simulink model "discrete_control_with_noise"  (Simulink 7.4)
settings: Solver=ode45  StartTime=0.0  StopTime=30.0  RelTol=1e-3
values from neighbouring files (symbols this model uses):
  f1 = (I_y-I_z)/I_x    [quadrocopter_param.m]
  f2 = rot.J_z/I_x    [quadrocopter_param.m]
  f3 = (I_z-I_x)/I_y    [quadrocopter_param.m]
  f4 = rot.J_z/I_y    [quadrocopter_param.m]
  f5 = (I_x-I_y)/I_z    [quadrocopter_param.m]
  g = 9.81    [quadrocopter_param.m]
  I_x = elec.I_x+bat.I_x+2*boom.I_1x+2*boom.I_1y+2*mot.I_1x+2*mot.I_1y+                             2*rot.I_1x+2*rot.I_1y    [quadrocopter_param.m]
  I_y = elec.I_y+bat.I_y+2*boom.I_1x+2*boom.I_1y+2*mot.I_1x+2*mot.I_1y+                             2*rot.I_1x+2*rot.I_1y    [quadrocopter_param.m]
  I_z = elec.I_z+bat.I_z+4*boom.I_1z+4*mot.I_1z+4*rot.I_1z    [quadrocopter_param.m]
  phi0 = 0.15    [Quadrocopter_control_Driver.m]    (also in calc_stability.m = 0; control_two_angles_Driver.m; control_two_angles_and_yawrate_Driver.m; discrete_control_phi_theta_rpsi_Driver.m)
  r_psi0 = 0    [Quadrocopter_control_Driver.m]    (also in calc_stability.m; control_two_angles_Driver.m = 0.01; control_two_angles_and_yawrate_Driver.m = 0.01; discrete_control_phi_theta_rpsi_Driver.m = 0.01)
  theta0 = 0.15    [Quadrocopter_control_Driver.m]    (also in calc_stability.m = 0; control_two_angles_Driver.m; control_two_angles_and_yawrate_Driver.m; discrete_control_phi_theta_rpsi_Driver.m)
  Ts = 0.005    [quadrocopter_param.m]
undefined symbols (not defined in the file or in its folder): boom
libraries: Copter_Library x5
settings Model: Creator=Robert  LastModifiedBy=roczit00

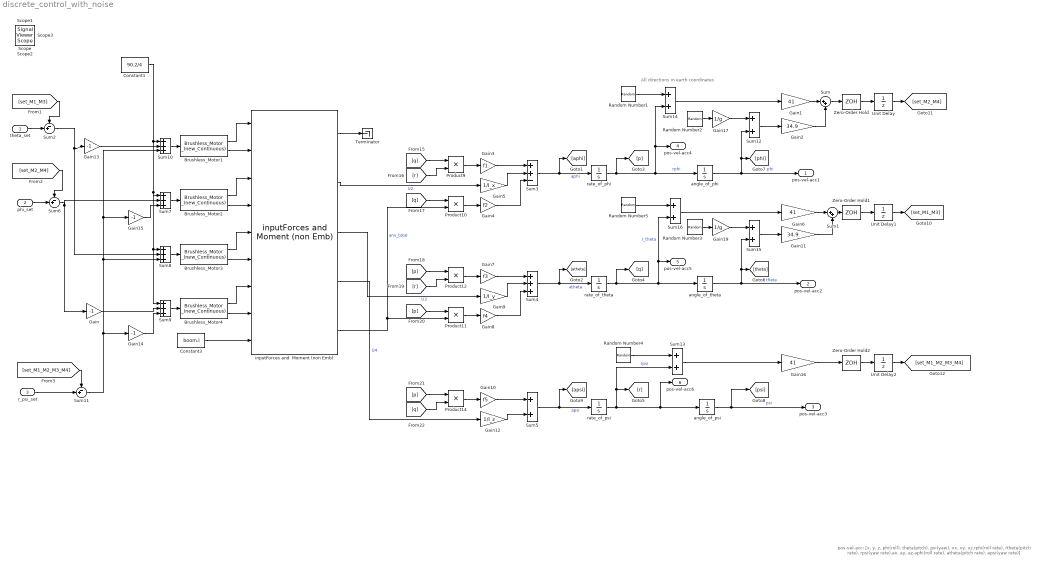
== system discrete_control_with_noise ==
  note: pos-vel-acc: [x, y, z, phi(roll), theta(pitch), psi(yaw), vx, vy, vz,rphi(roll rate), rtheta(pitch rate), rpsi(yaw rate),ax, ay, az,aphi(roll rate), atheta(pitch rate), apsi(yaw rate)]
  note: All directions in earth coordinates
  theta_set : Inport  OutDataType=fixdt(1, 16)  OutScaling=2^0
  phi_set : Inport  Port=2  OutDataType=fixdt(1, 16)  OutScaling=2^0
  r_psi_set : Inport  Port=3  OutDataType=fixdt(1, 16)  OutScaling=2^0
  Brushless_Motor{1..4} (4 alike) : Copter_Library/Brushless_Motor _(new_Continuous)  SystemSampleTime=-1  M_error=1
  Constant1 : Constant  Value=90.2/4  OutDataType=fixdt(1, 16)  OutScaling=2^0
  Constant3 : Constant  Value=boom.l  OutDataType=fixdt(1, 16)  OutScaling=2^0
  Gain{,13..15} (4 alike) : Gain  Gain=-1  ParameterDataType=fixdt(1, 16)  ParameterScaling=2^0  OutDataType=fixdt(1, 16)  OutScaling=2^0
  Gain1 : Gain  Gain=41  ParameterDataType=fixdt(1, 16)  ParameterScaling=2^0  OutDataType=fixdt(1, 16)  OutScaling=2^0
  Gain10 : Gain  Gain=f5  ParameterDataType=fixdt(1, 16)  ParameterScaling=2^0  OutDataType=fixdt(1, 16)  OutScaling=2^0
  Gain11 : Gain  Gain=34.9  ParameterDataType=fixdt(1, 16)  ParameterScaling=2^0  OutDataType=fixdt(1, 16)  OutScaling=2^0
  Gain12 : Gain  Gain=1/I_z  ParameterDataType=fixdt(1, 16)  ParameterScaling=2^0  OutDataType=fixdt(1, 16)  OutScaling=2^0
  Gain16 : Gain  Gain=41  ParameterDataType=fixdt(1, 16)  ParameterScaling=2^0  OutDataType=fixdt(1, 16)  OutScaling=2^0
  Gain17 : Gain  Gain=1/g  ParameterDataType=fixdt(1, 16)  ParameterScaling=2^0  OutDataType=fixdt(1, 16)  OutScaling=2^0
  Gain19 : Gain  Gain=1/g  ParameterDataType=fixdt(1, 16)  ParameterScaling=2^0  OutDataType=fixdt(1, 16)  OutScaling=2^0
  Gain2 : Gain  Gain=34.9  ParameterDataType=fixdt(1, 16)  ParameterScaling=2^0  OutDataType=fixdt(1, 16)  OutScaling=2^0
  Gain3 : Gain  Gain=f1  ParameterDataType=fixdt(1, 16)  ParameterScaling=2^0  OutDataType=fixdt(1, 16)  OutScaling=2^0
  Gain4 : Gain  Gain=f2  ParameterDataType=fixdt(1, 16)  ParameterScaling=2^0  OutDataType=fixdt(1, 16)  OutScaling=2^0
  Gain5 : Gain  Gain=1/I_x  ParameterDataType=fixdt(1, 16)  ParameterScaling=2^0  OutDataType=fixdt(1, 16)  OutScaling=2^0
  Gain6 : Gain  Gain=41  ParameterDataType=fixdt(1, 16)  ParameterScaling=2^0  OutDataType=fixdt(1, 16)  OutScaling=2^0
  Gain7 : Gain  Gain=f3  ParameterDataType=fixdt(1, 16)  ParameterScaling=2^0  OutDataType=fixdt(1, 16)  OutScaling=2^0
  Gain8 : Gain  Gain=f4  ParameterDataType=fixdt(1, 16)  ParameterScaling=2^0  OutDataType=fixdt(1, 16)  OutScaling=2^0
  Gain9 : Gain  Gain=1/I_y  ParameterDataType=fixdt(1, 16)  ParameterScaling=2^0  OutDataType=fixdt(1, 16)  OutScaling=2^0
  Product{9..12,14} (5 alike) : Product  OutDataType=fixdt(1, 16)  OutScaling=2^0  RndMeth=Zero
  Random Number1 : RandomNumber  Variance=3.0462e-8  Seed=45632  SampleTime=0.01
  Random Number2 : RandomNumber  Variance=0.0003  Seed=4564  SampleTime=0.01
  Random Number3 : RandomNumber  Variance=0.0003  Seed=676  SampleTime=Ts
  Random Number4 : RandomNumber  Variance=3.0462e-8  Seed=1634  SampleTime=0.01
  Random Number5 : RandomNumber  Variance=3.0462e-8  Seed=4731  SampleTime=0.01
  Sum : Sum  Inputs=|++  OutDataType=fixdt(1, 16)  OutScaling=2^0
  Sum1 : Sum  Inputs=|++  OutDataType=fixdt(1, 16)  OutScaling=2^0
  Sum{4,7..10} (5 alike) : Sum  Inputs=+++  OutDataType=fixdt(1, 16)  OutScaling=2^0
  Sum11 : Sum  Inputs=-+|  OutDataType=fixdt(1, 16)  OutScaling=2^0
  Sum{5,12..16} (6 alike) : Sum  OutDataType=fixdt(1, 16)  OutScaling=2^0
  Sum2 : Sum  Inputs=-+|  OutDataType=fixdt(1, 16)  OutScaling=2^0
  Sum3 : Sum  Inputs=++-  OutDataType=fixdt(1, 16)  OutScaling=2^0
  Sum6 : Sum  Inputs=-+|  OutDataType=fixdt(1, 16)  OutScaling=2^0
  Terminator : Terminator
  Unit Delay : UnitDelay  SampleTime=Ts
  Unit Delay1 : UnitDelay  SampleTime=Ts
  Unit Delay2 : UnitDelay  SampleTime=Ts
  Zero-Order Hold : ZeroOrderHold  SampleTime=Ts
  Zero-Order Hold1 : ZeroOrderHold  SampleTime=Ts
  Zero-Order Hold2 : ZeroOrderHold  SampleTime=Ts
  angle_of_phi : Integrator  InitialCondition=phi0
  angle_of_psi : Integrator
  angle_of_theta : Integrator  InitialCondition=theta0
  inputForces and  Moment (non Emb) : Copter_Library/inputForces and  Moment (non Emb)  SystemSampleTime=-1
  rate_of_phi : Integrator
  rate_of_psi : Integrator  InitialCondition=r_psi0
  rate_of_theta : Integrator
  pos-vel-acc1 : Outport  OutDataType=fixdt(1, 16)  OutScaling=2^0
  pos-vel-acc2 : Outport  Port=2  OutDataType=fixdt(1, 16)  OutScaling=2^0
  pos-vel-acc3 : Outport  Port=3  OutDataType=fixdt(1, 16)  OutScaling=2^0
  pos-vel-acc4 : Outport  Port=4  OutDataType=fixdt(1, 16)  OutScaling=2^0
  pos-vel-acc5 : Outport  Port=5  OutDataType=fixdt(1, 16)  OutScaling=2^0
  pos-vel-acc6 : Outport  Port=6  OutDataType=fixdt(1, 16)  OutScaling=2^0
  Scope : SignalViewerScope  IOType=viewer  ZoomMode=yonly  RefreshTime=0.035000
      settings: ShowLegends=on
  Scope1 : SignalViewerScope  IOType=viewer  ZoomMode=yonly  RefreshTime=0.035000
      settings: ShowLegends=on
  Scope2 : SignalViewerScope  IOType=viewer  ZoomMode=yonly  RefreshTime=0.035000
      settings: ShowLegends=on  SaveName=ScopeData2
  Scope3 : SignalViewerScope  IOType=viewer  ZoomMode=xonly  RefreshTime=0.035000
      settings: ShowLegends=on  SaveName=ScopeData3
  wires:
  Constant3/1 -> inputForces and  Moment (non Emb)/9
  Sum5/1 -> [apsi], rate_of_psi/1  "apsi"
  inputForces and  Moment (non Emb)/4 -> Gain12/1  "U4"
  Gain12/1 -> Sum5/2
  Gain10/1 -> Sum5/1
  Product14/1 -> Gain10/1
  [q] -> Product14/2
  [p] -> Product14/1
  Sum4/1 -> [atheta], rate_of_theta/1  "atheta"
  inputForces and  Moment (non Emb)/3 -> Gain9/1  "U3"
  Gain8/1 -> Sum4/3
  Gain9/1 -> Sum4/2
  Product11/1 -> Gain8/1
  [p] -> Product11/1
  Gain7/1 -> Sum4/1
  Product12/1 -> Gain7/1
  [r] -> Product12/2
  [p] -> Product12/1
  Sum3/1 -> [aphi], rate_of_phi/1  "aphi"
  Gain4/1 -> Sum3/3
  Gain5/1 -> Sum3/2
  inputForces and  Moment (non Emb)/2 -> Gain5/1  "U2"
  Product10/1 -> Gain4/1
  [q] -> Product10/1
  Gain3/1 -> Sum3/1
  Product9/1 -> Gain3/1
  [r] -> Product9/2
  [q] -> Product9/1
  inputForces and  Moment (non Emb)/5 -> Product11/2, Product10/2  "anv_total"
  angle_of_phi/1 -> pos-vel-acc1/1, [phi], Sum12/2  "phi"
  angle_of_theta/1 -> pos-vel-acc2/1, [theta], Sum15/2  "theta"
  angle_of_psi/1 -> [psi], pos-vel-acc3/1  "psi"
  rate_of_phi/1 -> [p], angle_of_phi/1, pos-vel-acc4/1, Sum14/2  "rphi"
  rate_of_theta/1 -> angle_of_theta/1, pos-vel-acc5/1, Sum16/2, [q]  "r_theta"
  rate_of_psi/1 -> angle_of_psi/1, pos-vel-acc6/1, [r], Sum13/2  "rpsi"
  Brushless_Motor1/1 -> inputForces and  Moment (non Emb)/1
  Brushless_Motor1/2 -> inputForces and  Moment (non Emb)/2
  Brushless_Motor2/1 -> inputForces and  Moment (non Emb)/3
  Brushless_Motor2/2 -> inputForces and  Moment (non Emb)/4
  Brushless_Motor3/1 -> inputForces and  Moment (non Emb)/5
  Brushless_Motor3/2 -> inputForces and  Moment (non Emb)/6
  Brushless_Motor4/1 -> inputForces and  Moment (non Emb)/7
  Brushless_Motor4/2 -> inputForces and  Moment (non Emb)/8
  Gain1/1 -> Sum/1
  Gain2/1 -> Sum/2
  Gain6/1 -> Sum1/1
  Gain11/1 -> Sum1/2
  [set_M1_M3] -> Sum2/1
  theta_set/1 -> Sum2/2
  Sum2/1 -> Gain13/1, Sum8/2
  phi_set/1 -> Sum6/2
  [set_M2_M4] -> Sum6/1
  Sum6/1 -> Gain/1, Sum7/2
  inputForces and  Moment (non Emb)/1 -> Terminator/1
  Sum9/1 -> Brushless_Motor4/1
  Sum8/1 -> Brushless_Motor3/1
  Sum7/1 -> Brushless_Motor2/1
  Sum10/1 -> Brushless_Motor1/1
  Constant1/1 -> Sum10/1, Sum7/1, Sum8/1, Sum9/1
  Gain13/1 -> Sum10/2
  Gain/1 -> Sum9/2
  r_psi_set/1 -> Sum11/2
  [set_M1_M2_M3_M4] -> Sum11/1
  Gain15/1 -> Sum7/3
  Sum11/1 -> Gain14/1, Sum8/3, Gain15/1, Sum10/3
  Gain14/1 -> Sum9/3
  Sum/1 -> Zero-Order Hold/1
  Sum1/1 -> Zero-Order Hold1/1
  Gain16/1 -> Zero-Order Hold2/1
  Zero-Order Hold2/1 -> Unit Delay2/1
  Unit Delay2/1 -> [set_M1_M2_M3_M4]
  Zero-Order Hold1/1 -> Unit Delay1/1
  Unit Delay1/1 -> [set_M1_M3]
  Zero-Order Hold/1 -> Unit Delay/1
  Unit Delay/1 -> [set_M2_M4]
  Random Number2/1 -> Gain17/1
  Gain17/1 -> Sum12/1
  Random Number1/1 -> Sum14/1
  Sum14/1 -> Gain1/1
  Sum12/1 -> Gain2/1
  Random Number3/1 -> Gain19/1
  Gain19/1 -> Sum15/1
  Sum15/1 -> Gain11/1
  Sum16/1 -> Gain6/1
  Random Number5/1 -> Sum16/1
  Sum13/1 -> Gain16/1
  Random Number4/1 -> Sum13/1
